simulink model "sDynSys"  (Simulink 7.9)
settings: Solver=ode23s  StartTime=0.0  StopTime=10  FixedStep=0.2  RelTol=1e-6
settings Model: Creator=Roger  LastModifiedBy=rskjetne
settings OptimizationCC: InitFltsAndDblsToZero=on
settings DebuggingCC: SaveWithParameterizedLinksMsg=none  SignalResolutionControl=TryResolveAllWithWarning  MultiTaskDSMMsg=warning  MultiTaskCondExecSysMsg=none  FcnCallInpInsideContextMsg=Use local settings  StrictBusMsg=None
settings RTWCC: IncludeERTFirstTime=on
settings GRTTargetCC: TargetFcnLib=ansi_tfl_tmw.mat  CombineOutputUpdateFcns=off  GRTInterface=on

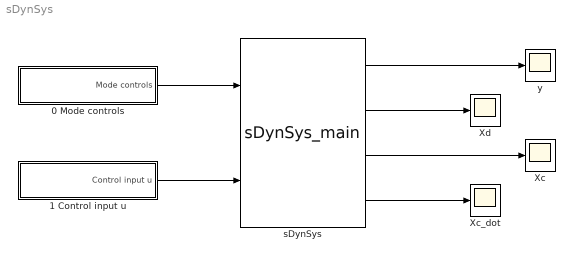
== system sDynSys ==
  0 Mode controls : Subsystem
  1 Control input u : Subsystem
  Xc : Scope
      settings: TimeRange=50  YMin=-10  YMax=50  SaveName=xc
  Xc_dot : Scope
      settings: TimeRange=10  YMin=-2500  YMax=500  SaveName=xc_dot
  Xd : Scope
      settings: TimeRange=20  SaveName=xd
  sDynSys : S-Function  FunctionName=sDynSys_main  Parameters=SimParam, Fname, Xc0, Xd0  EnableBusSupport=off
  y : Scope
      settings: TimeRange=10  YMin=-1.5  YMax=1.5  SaveName=y
  wires:
  0 Mode controls/1(Mode controls) -> sDynSys/1
  1 Control input u/1(Control input u) -> sDynSys/2
  sDynSys/1 -> y/1
  sDynSys/2 -> Xd/1
  sDynSys/3 -> Xc/1
  sDynSys/4 -> Xc_dot/1

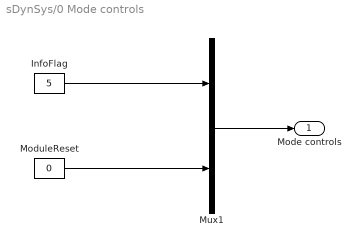
== system sDynSys/0 Mode controls ==
  InfoFlag : Constant  Value=5
  ModuleReset : Constant  Value=0
  Mux1 : Mux  Inputs=2
  Mode controls : Outport
  wires:
  InfoFlag/1 -> Mux1/1
  Mux1/1 -> Mode controls/1
  ModuleReset/1 -> Mux1/2

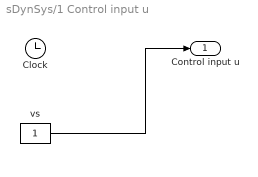
== system sDynSys/1 Control input u ==
  Clock : Clock
  vs : Constant
  Control input u : Outport
  wires:
  vs/1 -> Control input u/1
